simulink library "lib_ESS"  (R2018b)
settings: Solver=VariableStepAuto  StartTime=0.0  StopTime=10.0  RelTol=1e-3
undefined symbols (not defined in the file or in its folder): A123_ESS, C1, C2, DiscIntNeverNeededParam, R0, R1, R2, soc_bpt, t_step
settings Model: Creator=amankalia  LastModifiedBy=Aman-Home

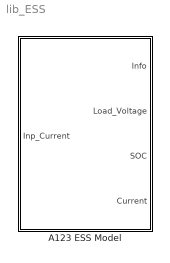
== system lib_ESS ==
  A123 ESS Model : Subsystem  mask{Q_max_cell=A123_ESS.Q_cell_max_Ah, Np=A123_ESS.Np, Ns=A123_ESS.Ns, Nmod=A123_ESS.Nmod, soc_init=A123_ESS.Init_soc, soc_bpt=soc_bpt, R0=R0, R1=R1, C1=C1, R2=R2, C2=C2, t_step=t_step}
      mask prompts: Q_max_cell "Max cell capacity [Ah]:"; Np "Number of cells in parallel []:"; Ns "Numer of cells in series []:"; Nmod "Number of modules []:"; soc_init "Initial SoC/100 []:"; soc_bpt "SoC break points []:"; R0 "Internal resistance vector []:"; R1 "RC1 resistance vector []:"; C1 "RC1 capacitance vector []:"; R2 "RC2 resistance vector []:"; C2 "RC2 capacitance vector []:"; t_step "Simulation time step:"
      mask DialogControl DescGroupVar Prompt: Parameter Settings
      mask DialogControl DescTextVar Prompt: This model emulates an A123 ESS used by UW EcoCAR Team.
      mask DialogControl BatParamGroupVar Prompt: Battery Parameters
      mask DialogControl EstParamGroupVar Prompt: Estimated RC Parameters
      mask DialogControl MiscSettGroupVar Prompt: Miscellaneous Settings

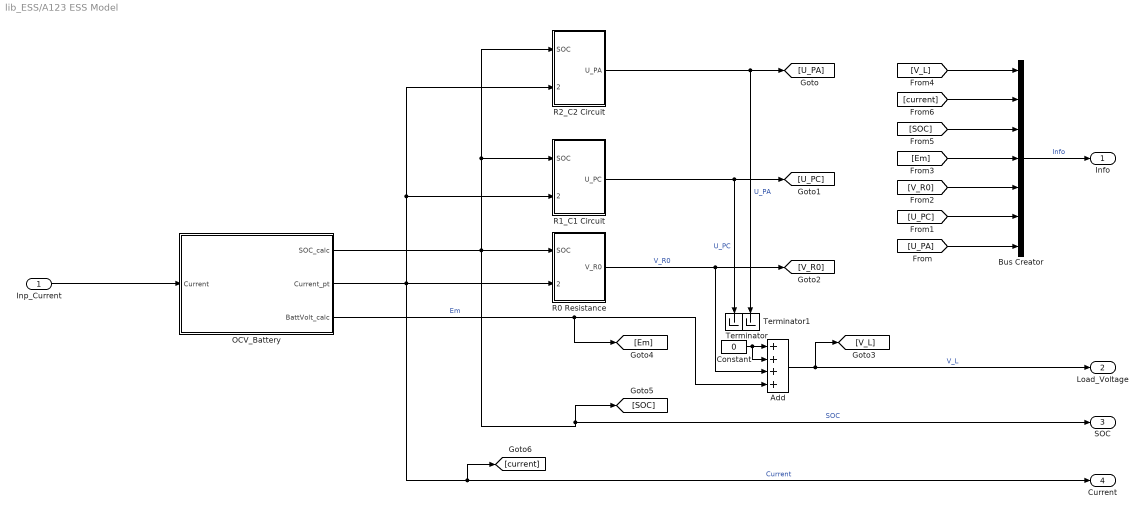
== system lib_ESS/A123 ESS Model ==
  Inp_Current : Inport
  Add : Sum  Inputs=++++
  Bus Creator : BusCreator  Inputs=7
  Constant : Constant  Value=0
  OCV_Battery : Subsystem
  R0 Resistance : Subsystem
  R1_C1 Circuit : Subsystem
  R2_C2 Circuit : Subsystem
  Terminator : Terminator
  Terminator1 : Terminator
  Info : Outport
  Load_Voltage : Outport  Port=2
  SOC : Outport  Port=3
  Current : Outport  Port=4
  wires:
  Constant/1 -> Add/1, Add/2
  [V_L] -> Bus Creator/1
  Bus Creator/1 -> Info/1  "Info"
  [V_R0] -> Bus Creator/5
  OCV_Battery/3(BattVolt_calc) -> Add/4, [Em]  "Em"
  [U_PC] -> Bus Creator/6
  R1_C1 Circuit/1(U_PC) -> [U_PC], Terminator/1  "U_PC"
  OCV_Battery/1(SOC_calc) -> R0 Resistance/1(SOC), R1_C1 Circuit/1(SOC), R2_C2 Circuit/1(SOC), [SOC], SOC/1  "SOC"
  OCV_Battery/2(Current_pt) -> R0 Resistance/2(Current), R1_C1 Circuit/2(Current), R2_C2 Circuit/2(Current), [current], Current/1  "Current"
  R2_C2 Circuit/1(U_PA) -> [U_PA], Terminator1/1  "U_PA"
  R0 Resistance/1(V_R0) -> Add/3, [V_R0]  "V_R0"
  [Em] -> Bus Creator/4
  Add/1 -> [V_L], Load_Voltage/1  "V_L"
  [current] -> Bus Creator/2
  Inp_Current/1 -> OCV_Battery/1(Current)
  [U_PA] -> Bus Creator/7
  [SOC] -> Bus Creator/3

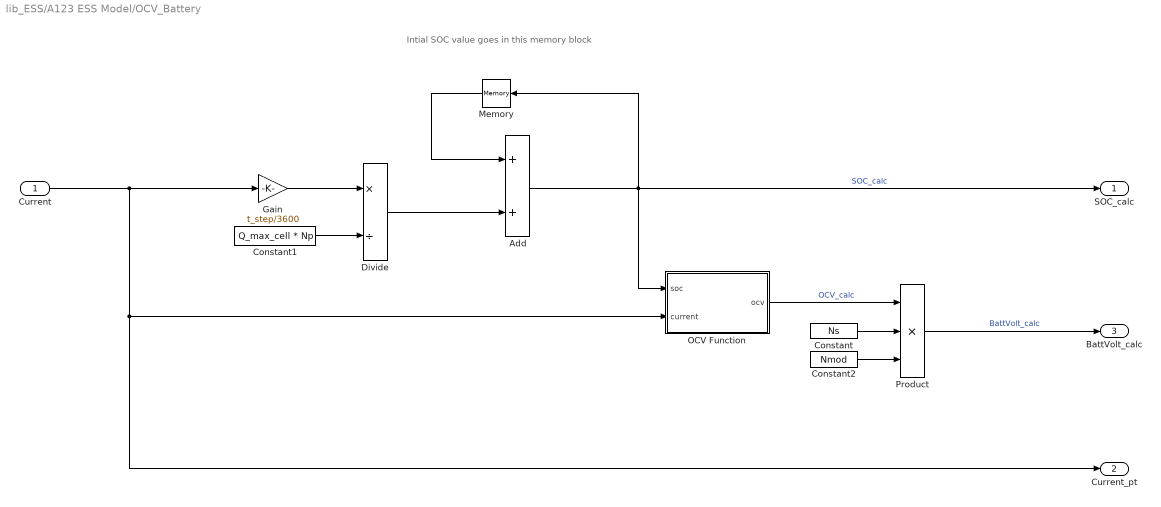
== system lib_ESS/A123 ESS Model/OCV_Battery ==
  note: Intial SOC value goes in this memory block
  Current : Inport
  Add : Sum
  Constant : Constant  Value=Ns
  Constant1 : Constant  Value=Q_max_cell * Np
  Constant2 : Constant  Value=Nmod
  Divide : Product  Inputs=*/
  Gain : Gain  Gain=t_step/3600
  Memory : Memory  InitialCondition=soc_init  InheritSampleTime=on  LinearizeAsDelay=on
  OCV Function : MATLAB Function  TreatAsAtomicUnit=on
  Product : Product  Inputs=3
  SOC_calc : Outport
  Current_pt : Outport  Port=2
  BattVolt_calc : Outport  Port=3
  wires:
  Product/1 -> BattVolt_calc/1  "BattVolt_calc"
  Divide/1 -> Add/2
  Constant/1 -> Product/2
  Add/1 -> Memory/1, OCV Function/1(soc), SOC_calc/1  "SOC_calc"
  Constant1/1 -> Divide/2
  OCV Function/1(ocv) -> Product/1  "OCV_calc"
  Constant2/1 -> Product/3
  Memory/1 -> Add/1
  Gain/1 -> Divide/1
  Current/1 -> Gain/1, Current_pt/1, OCV Function/2(current)

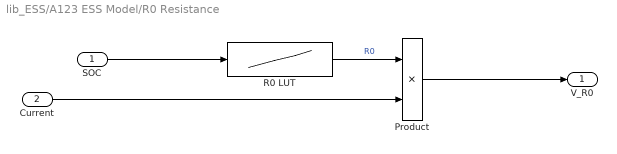
== system lib_ESS/A123 ESS Model/R0 Resistance ==
  SOC : Inport
  Current : Inport  Port=2
  Product : Product
  R0 LUT : Lookup_n-D  NumberOfTableDimensions=1  BreakpointsForDimension1=soc_bpt  Table=R0  InternalRulePriority=Speed  RndMeth=Simplest  InputSameDT=on
  V_R0 : Outport
  wires:
  Product/1 -> V_R0/1
  Current/1 -> Product/2
  SOC/1 -> R0 LUT/1
  R0 LUT/1 -> Product/1  "R0"

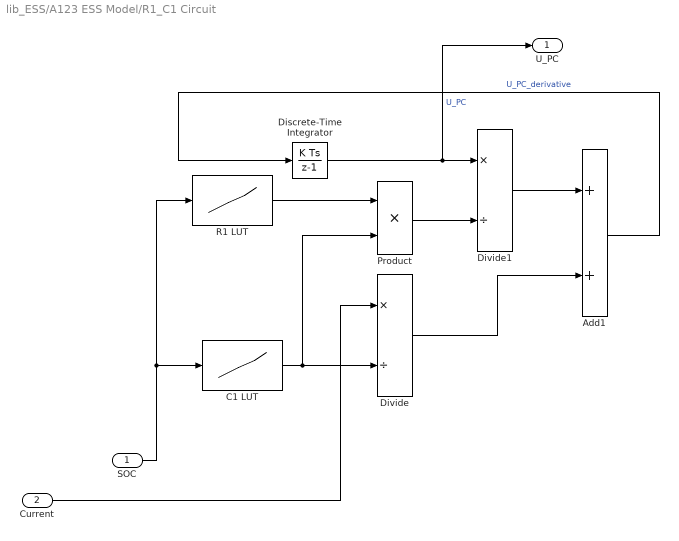
== system lib_ESS/A123 ESS Model/R1_C1 Circuit ==
  SOC : Inport
  Current : Inport  Port=2
  Add1 : Sum
  C1 LUT : Lookup_n-D  NumberOfTableDimensions=1  BreakpointsForDimension1=soc_bpt  Table=C1  InternalRulePriority=Speed  RndMeth=Simplest  InputSameDT=on
  Discrete-Time Integrator : DiscreteIntegrator  SampleTime=-1  ICPrevOutput=DiscIntNeverNeededParam  ICPrevScaledInput=DiscIntNeverNeededParam
  Divide : Product  Inputs=*/
  Divide1 : Product  Inputs=*/
  Product : Product
  R1 LUT : Lookup_n-D  NumberOfTableDimensions=1  BreakpointsForDimension1=soc_bpt  Table=R1  InternalRulePriority=Speed  RndMeth=Simplest  InputSameDT=on
  U_PC : Outport
  wires:
  Current/1 -> Divide/1
  Add1/1 -> Discrete-Time Integrator/1  "U_PC_derivative"
  Discrete-Time Integrator/1 -> Divide1/1, U_PC/1  "U_PC"
  R1 LUT/1 -> Product/1
  Divide/1 -> Add1/2
  C1 LUT/1 -> Divide/2, Product/2
  Divide1/1 -> Add1/1
  SOC/1 -> C1 LUT/1, R1 LUT/1
  Product/1 -> Divide1/2

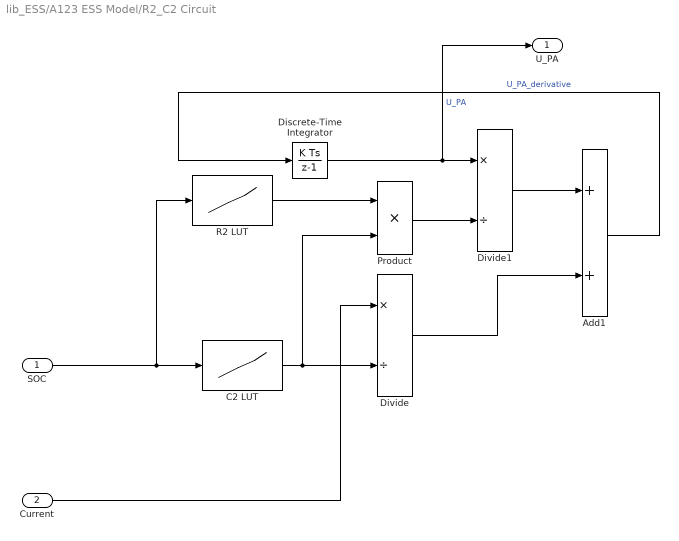
== system lib_ESS/A123 ESS Model/R2_C2 Circuit ==
  SOC : Inport
  Current : Inport  Port=2
  Add1 : Sum
  C2 LUT : Lookup_n-D  NumberOfTableDimensions=1  BreakpointsForDimension1=soc_bpt  Table=C2  InternalRulePriority=Speed  RndMeth=Simplest  InputSameDT=on
  Discrete-Time Integrator : DiscreteIntegrator  SampleTime=-1  ICPrevOutput=DiscIntNeverNeededParam  ICPrevScaledInput=DiscIntNeverNeededParam
  Divide : Product  Inputs=*/
  Divide1 : Product  Inputs=*/
  Product : Product
  R2 LUT : Lookup_n-D  NumberOfTableDimensions=1  BreakpointsForDimension1=soc_bpt  Table=R2  InternalRulePriority=Speed  RndMeth=Simplest  InputSameDT=on
  U_PA : Outport
  wires:
  Current/1 -> Divide/1
  Add1/1 -> Discrete-Time Integrator/1  "U_PA_derivative"
  Discrete-Time Integrator/1 -> Divide1/1, U_PA/1  "U_PA"
  R2 LUT/1 -> Product/1
  Divide/1 -> Add1/2
  C2 LUT/1 -> Divide/2, Product/2
  Divide1/1 -> Add1/1
  SOC/1 -> C2 LUT/1, R2 LUT/1
  Product/1 -> Divide1/2

== matlab function lib_ESS/A123 ESS Model/OCV_Battery/OCV Function ==
  data: soc input; ocv output; current input
function ocv = fcn(soc, current)

if current < 0
    %% 0-20 Model Fit
    if (soc <= 0.2)
        ocv = 3.17*exp(0.1*soc) - 2.76*exp(-65.25*soc);
    %% 20-80 Model Fit
    elseif (soc > 0.2 && soc <= 0.8)
        ocv = 0.165*soc + 3.20;
    %% 80-100 Model Fit
    else
        ocv = 0.2*(soc^74.2) + 3.33;
    end
else
    %% 0-20 Model Fit
    if (soc <= 0.2)
        ocv = 3.19*exp(0.098*soc) - 1.09*exp(-48.81*soc);
    %% 20-80 Model Fit
    elseif (soc > 0.2 && soc <= 0.8)
        ocv = 0.148*soc + 3.222;
    %% 80-100 Model Fit
    else
        ocv = 0.336*(soc^108.2) + 3.34;
    end
end
